simulink model "climb_h1500"  (R2023b)
settings: Solver=VariableStepAuto  StartTime=0.0  StopTime=10  RelTol=1e-3
undefined symbols (not defined in the file or in its folder): climb_h1500
settings Model: Creator=阿汪  LastModifiedBy=阿汪

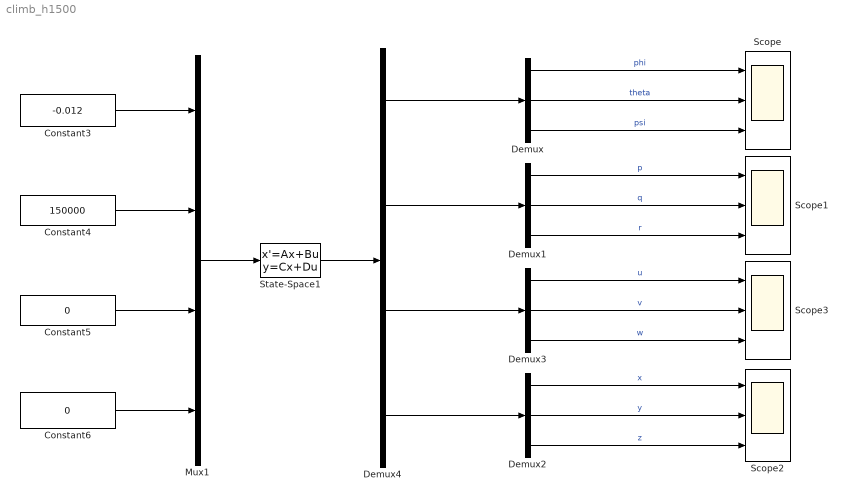
== system climb_h1500 ==
  Constant3 : Constant  Value=-0.012
  Constant4 : Constant  Value=150000
  Constant5 : Constant  Value=0
  Constant6 : Constant  Value=0
  Demux{,1..3} (4 alike) : Demux  Outputs=3
  Demux4 : Demux
  Mux1 : Mux
  Scope{,1..3} (4 alike) : Scope  NumInputPorts=3
  State-Space1 : StateSpace  A=climb_h1500.A  B=climb_h1500.B  C=climb_h1500.C  D=climb_h1500.D  InitialCondition=[0;0.1;0;0;-0.02;0;130;0;8;0;0;-1500]
  wires:
  Demux4/1 -> Demux/1
  Demux1/2 -> Scope1/2  "q"
  Demux/3 -> Scope/3  "psi"
  Demux1/1 -> Scope1/1  "p"
  Demux3/2 -> Scope3/2  "v"
  Constant5/1 -> Mux1/3
  Demux3/3 -> Scope3/3  "w"
  Mux1/1 -> State-Space1/1
  Demux1/3 -> Scope1/3  "r"
  Demux2/3 -> Scope2/3  "z"
  Constant4/1 -> Mux1/2
  Demux3/1 -> Scope3/1  "u"
  Constant6/1 -> Mux1/4
  Demux4/2 -> Demux1/1
  Demux2/2 -> Scope2/2  "y"
  Demux/2 -> Scope/2  "theta"
  Demux4/3 -> Demux3/1
  Demux4/4 -> Demux2/1
  State-Space1/1 -> Demux4/1
  Demux2/1 -> Scope2/1  "x"
  Demux/1 -> Scope/1  "phi"
  Constant3/1 -> Mux1/1
